simulink model "TEST_C___MAPD"  (R2015b)
settings: Solver=ode23tb  StartTime=0.0  StopTime=1  RelTol=1e-3
InitFcn:
  | eps=1e-10
  | 
  | Lg=90e-6;
  | l=100e-6; r=2e-3;
  | tff=10e-6;
  | w=2*pi*60;
  | z_lead =966.3602;
  | p_lead =5.6324e+03;
  | Vdc=2000;
undefined symbols (not defined in the file or in its folder): C, magnitude
libraries: powerlib x26, powerlib_meascontrol x12, simulink x8, simulink_extras x3
settings Model: Creator=Shahed Mortazavian  LastModifiedBy=Masoud
settings DataIOCC: SaveFormat=Array  SignalLoggingSaveFormat=ModelDataLogs
settings OptimizationCC: ExpressionDepthLimit=2147483647
settings DebuggingCC: UnderspecifiedInitializationDetection=Classic  MergeDetectMultiDrivingBlocksExec=none  SolverPrmCheckMsg=warning  FcnCallInpInsideContextMsg=UseLocalSettings  StateNameClashWarn=warning
settings HardwareCC: ProdBitPerPointer=32  ProdLargestAtomicFloat=None  ProdIntDivRoundTo=Undefined  ProdEndianess=Unspecified  ProdWordSize=32  ProdHWDeviceType=32-bit Generic
settings GRTTargetCC: GeneratePreprocessorConditionals=Disable all  CombineOutputUpdateFcns=off  GRTInterface=on
settings ConfigComp: CovModelRefEnable=Off  CovSFcnEnable=off

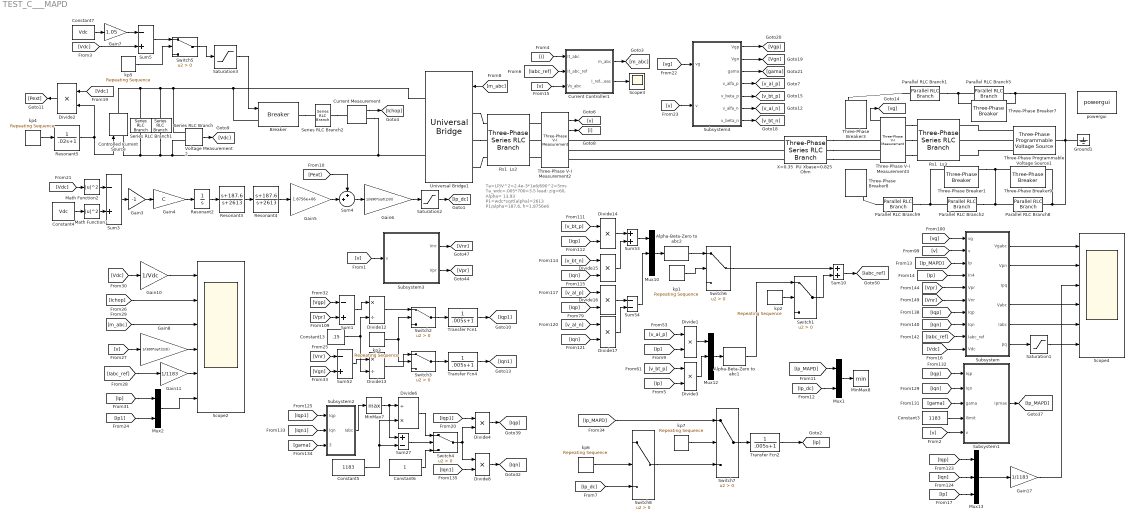
== system TEST_C___MAPD ==
  note: Ta=LP/V^2=2.4e-3*1e6/690^2=5ms
      | Ta_wdc=.005*700=3.5
      | lead: zig=60, Alpha= 13.93
      | P1=wdc*sqrt(alpha)=2613
      | P1/alpha=187.6, h=1.8756e6
  Alpha-Beta-Zero to abc1 : powerlib_meascontrol/Transformations/Alpha-Beta-Zero to abc
  Alpha-Beta-Zero to abc2 : powerlib_meascontrol/Transformations/Alpha-Beta-Zero to abc
  Breaker : powerlib/Elements/Breaker  InitialState=0  SwitchingTimes="[1/60  5/60]"  External=on  BreakerResistance=0.01  SnubberResistance=1e6  SnubberCapacitance=inf  Measurements=None  MoreParameters=on  NoBreakLoop=off
  Constant13 : Constant  Value=.15
  Constant3 : Constant  Value=1183
  Constant4 : Constant  Value=Vdc
  Constant5 : Constant  Value=1183
  Constant6 : Constant
  Constant7 : Constant  Value=Vdc
  Controlled Current Source : powerlib/Electrical Sources/Controlled Current Source  Initialize=on  Source_Type=AC  Amplitude=0  Phase=0  Frequency=0  Measurements=None
  Current Controller1 : Subsystem
  Current Measurement : powerlib/Measurements/Current Measurement  PhasorSimulation=off  OutputType=Complex  PSBequivalent=0
  Divide{1..4,8,14..17} (9 alike) : Product  Inputs=**
  Divide12 : Product  Inputs=*/
  Divide13 : Product  Inputs=*/
  Divide6 : Product  Inputs=/*
  Gain10 : Gain  Gain=1/Vdc
  Gain11 : Gain  Gain=1/1183
  Gain17 : Gain  Gain=1/1183
  Gain3 : Gain  Gain=-1
  Gain4 : Gain  Gain=C
  Gain5 : Gain  Gain=1.8756e+06
  Gain6 : Gain  Gain=1/(690*sqrt(2/3))
  Gain7 : Gain  Gain=1.05
  Gain8 : Gain  Gain=1/(690*sqrt(2/3))
  Ground1 : powerlib/Elements/Ground  LConnTagsString=a
  Math Function1 : Math  Operator=magnitude^2  SaturateOnIntegerOverflow=on
  Math Function2 : Math  Operator=magnitude^2  SaturateOnIntegerOverflow=on
  MinMax7 : MinMax  Function=max
  MinMax8 : MinMax
  Mux1 : Mux  Inputs=2
  Mux10 : Mux  Inputs=3
  Mux12 : Mux  Inputs=3
  Mux13 : Mux  Inputs=3
  Mux2 : Mux  Inputs=2
  Parallel RLC Branch1 : powerlib/Elements/Parallel RLC Branch  LConnTagsString=a  RConnTagsString=__new0  BranchType=R  Resistance=1e-3  Inductance=1e-3  SetiL0=off  InitialCurrent=0  Capacitance=1e-6  Setx0=off  InitialVoltage=0  Measurements=None
  Parallel RLC Branch2 : powerlib/Elements/Parallel RLC Branch  LConnTagsString=a  RConnTagsString=__new0  BranchType=R  Resistance=1e-3  Inductance=1e-3  SetiL0=off  InitialCurrent=0  Capacitance=1e-6  Setx0=off  InitialVoltage=0  Measurements=None
  Parallel RLC Branch5 : powerlib/Elements/Parallel RLC Branch  LConnTagsString=a  RConnTagsString=__new0  BranchType=R  Resistance=.3e-3  Inductance=1e-3  SetiL0=off  InitialCurrent=0  Capacitance=1e-6  Setx0=off  InitialVoltage=0  Measurements=None
  Parallel RLC Branch8 : powerlib/Elements/Parallel RLC Branch  LConnTagsString=a  RConnTagsString=__new0  BranchType=R  Resistance=1e-3  Inductance=1e-3  SetiL0=off  InitialCurrent=0  Capacitance=1e-6  Setx0=off  InitialVoltage=0  Measurements=None
  Parallel RLC Branch9 : powerlib/Elements/Parallel RLC Branch  LConnTagsString=a  RConnTagsString=__new0  BranchType=R  Resistance=2e-3  Inductance=1e-3  SetiL0=off  InitialCurrent=0  Capacitance=1e-6  Setx0=off  InitialVoltage=0  Measurements=None
  Resonant2 : TransferFcn  Denominator=[1 0 ]
  Resonant3 : TransferFcn  Numerator=[1 187.6]  Denominator=[1 2613]
  Resonant4 : TransferFcn  Numerator=[1 187.6]  Denominator=[1 2613]
  Resonant5 : TransferFcn  Denominator=[.02 1]
  Rs1  Ls2 : powerlib/Elements/Three-Phase Series RLC Branch  LConnTagsString=A|B|C  RConnTagsString=A|B|C  BranchType=RL  Resistance=r  Inductance=l  Capacitance=1e-6  Measurements=None
  Rs1  Ls3 : powerlib/Elements/Three-Phase Series RLC Branch  LConnTagsString=A|B|C  RConnTagsString=A|B|C  BranchType=R  Resistance=1e-3  Inductance=l  Capacitance=1e-6  Measurements=None
  Saturation1 : Saturate  UpperLimit=1.5  LowerLimit=-.5
  Saturation2 : Saturate  UpperLimit=2000  LowerLimit=0
  Saturation3 : Saturate  UpperLimit=1000  LowerLimit=0
  Scope2 : Scope  NumInputPorts=6
  Scope3 : Scope
  Scope4 : Scope  NumInputPorts=6
  Series RLC Branch : powerlib/Elements/Series RLC Branch  LConnTagsString=__new0  RConnTagsString=__new0  BranchType=C  Resistance=1  Inductance=1e-3  SetiL0=off  InitialCurrent=0  Capacitance=C*2  Setx0=on  InitialVoltage=Vdc  Measurements=None
  Series RLC Branch1 : powerlib/Elements/Series RLC Branch  LConnTagsString=__new0  RConnTagsString=__new0  BranchType=R  Resistance=1e10  Inductance=1e-3  SetiL0=off  InitialCurrent=0  Capacitance=C  Setx0=on  InitialVoltage=2500  Measurements=None
  Series RLC Branch2 : powerlib/Elements/Series RLC Branch  LConnTagsString=__new0  RConnTagsString=__new0  BranchType=R  Resistance=1  Inductance=1e-3  SetiL0=off  InitialCurrent=0  Capacitance=C  Setx0=on  InitialVoltage=2500  Measurements=None
  Subsystem : Subsystem
  Subsystem1 : Subsystem
  Subsystem2 : Subsystem
  Subsystem3 : Subsystem
  Subsystem4 : Subsystem
  Sum{1,3,5,52} (4 alike) : Sum  Inputs=-+
  Sum10 : Sum
  Sum27 : Sum  Inputs=+-
  Sum4 : Sum  Inputs=++|
  Sum53 : Sum
  Sum54 : Sum  Inputs=--
  Switch{1..8} (8 alike) : Switch  Criteria=u2 > Threshold
  Three-Phase Programmable Voltage Source1 : powerlib/Electrical Sources/Three-Phase Programmable Voltage Source  PositiveSequence=[690 0 60]  VariationEntity=Amplitude  VariationType=Table of time-amplitude pairs  VariationTypeAlt=Step  VariationStep=0.5  VariationRate=10  VariationMagnitude=0.3  VariationFrequency=2  VariationTiming=[1 2]  VariationPhaseA=on  Amplitudes=[1 1 .61 .61]  TimeValues=[0 .3 .30001 10]  HarmonicGeneration=off  HarmonicA=[3 0.2 -25 0]  HarmonicB=[2 0.15 35 2]  Timing="[0.05  3]"  BusType=swing  Pref=0  Qref=0  Qmin=-inf  Qmax=inf
  Three-Phase V-I Measurement2 : powerlib/Measurements/Three-Phase V-I Measurement  VoltageMeasurement=phase-to-ground  SetLabelV=off  LabelV=Vabc  Vpu=off  VpuLL=off  CurrentMeasurement=yes  SetLabelI=off  LabelI=Iabc  Ipu=off  Pbase=100e6  Vbase=500e3  OutputType=Complex  PhasorSimulation=off  PSBequivalent=0
  Three-Phase V-I Measurement3 : powerlib/Measurements/Three-Phase V-I Measurement  VoltageMeasurement=phase-to-ground  SetLabelV=off  LabelV=Vabc  Vpu=off  VpuLL=off  CurrentMeasurement=yes  SetLabelI=off  LabelI=Iabc  Ipu=off  Pbase=100e6  Vbase=500e3  OutputType=Complex  PhasorSimulation=off  PSBequivalent=0
  Three-Phase Breaker1 : powerlib/Elements/Three-Phase Breaker  InitialState=open  SwitchA=on  SwitchB=on  SwitchC=on  SwitchTimes=.6  External=off  BreakerResistance=1e-40  SnubberResistance=1e6  SnubberCapacitance=inf  Measurements=None
  Three-Phase Breaker3 : powerlib/Elements/Three-Phase Breaker  InitialState=open  SwitchA=on  SwitchB=on  SwitchC=on  SwitchTimes=.3  External=off  BreakerResistance=1e-40  SnubberResistance=1e6  SnubberCapacitance=inf  Measurements=None
  Three-Phase Breaker7 : powerlib/Elements/Three-Phase Breaker  InitialState=open  SwitchA=on  SwitchB=on  SwitchC=on  SwitchTimes=.5  External=off  BreakerResistance=1e-40  SnubberResistance=1e6  SnubberCapacitance=inf  Measurements=None
  Three-Phase Breaker8 : powerlib/Elements/Three-Phase Breaker  InitialState=open  SwitchA=on  SwitchB=on  SwitchC=on  SwitchTimes=.2  External=off  BreakerResistance=1e-40  SnubberResistance=1e6  SnubberCapacitance=inf  Measurements=None
  Three-Phase Breaker9 : powerlib/Elements/Three-Phase Breaker  InitialState=open  SwitchA=on  SwitchB=on  SwitchC=on  SwitchTimes=.6  External=off  BreakerResistance=1e-40  SnubberResistance=1e6  SnubberCapacitance=inf  Measurements=None
  Transfer Fcn1 : TransferFcn  Numerator=1  Denominator=[.005 1]
  Transfer Fcn2 : TransferFcn  Numerator=1  Denominator=[.005 1]
  Transfer Fcn4 : TransferFcn  Numerator=1  Denominator=[.005 1]
  Universal Bridge1 : powerlib/Power Electronics/Universal Bridge  Arms=3  SnubberResistance=1e5  SnubberCapacitance=inf  Device=Average-model based VSC  Ron=1e-3  Lon=0  ForwardVoltages="[  0  0  ]"  ForwardVoltage=0  GTOparameters=[ 10e-6 , 20e-6 ]  IGBTparameters=[ 1e-6 , 2e-6 ]  Measurements=None  Measurements_2=None  converterType=Rectifier
  Voltage Measurement2 : powerlib/Measurements/Voltage Measurement  PhasorSimulation=off  OutputType=Complex  PSBequivalent=0
  X=0.35  PU Xbase=0.825  Ohm : powerlib/Elements/Three-Phase Series RLC Branch  LConnTagsString=A|B|C  RConnTagsString=A|B|C  BranchType=L  Resistance=.0001  Inductance=.15/377  Capacitance=1e-6  Measurements=None
  kp1 : simulink/Sources/Repeating Sequence  rep_seq_t=[0 .3 .3+eps 10]  rep_seq_y=[0 0 1 1]
  kp2 : simulink/Sources/Repeating Sequence  rep_seq_t=[0 .03 .03+eps 10]  rep_seq_y=[0 0 1 1]
  kp3 : simulink/Sources/Repeating Sequence  rep_seq_t=[0 .31 .31+eps 10]  rep_seq_y=[0 0 1 1]
  kp4 : simulink/Sources/Repeating Sequence  rep_seq_t=[0 .02 .02+eps 10]  rep_seq_y=3/2*400*[0 0 .8 .8]
  kp5 : simulink/Sources/Repeating Sequence  rep_seq_t=[0 .3 .3+eps 10]  rep_seq_y=[0 0 1 1]
  kp6 : simulink/Sources/Repeating Sequence  rep_seq_t=[0 .5 .5+eps 10]  rep_seq_y=[0 0 1 1]
  kp7 : simulink/Sources/Repeating Sequence  rep_seq_t=[0 .7 .7+eps 10]  rep_seq_y=[0 0 1 1]
  powergui : powerlib/powergui  Priority=2  SimulationMode=Discrete  SolverType=Tustin  SampleTime=5e-5  frequency=60  SPID=off  DisableSnubberDevices=off  DisableRonSwitches=off  DisableVfSwitches=off  SwTol=0  DisplayEquations=off  Interpol=off  ExternalGateDelay=off  methode=off  Ts=0  FunctionMessages=off  echomessages=off  HookPort=off  EnableUseOfTLC=off  x0status=blocks  frequencyindice=0  Pbase=100e6  ErrMax=1e-4  Iterations=50  UnitsV=kV  UnitsW=MW  buscounter=0  RestoreLinks=warning  ResistiveCurrentMeasurement=off  Frange=[0:2:500]  Ylog=off  Xlog=on  ShowGrid=off  save=off  variable=ZData  structure=Data  ZoomFFT=off  StartTime=.22  cycles=2  DisplayStyle=1  fundamental=60  FreqAxis=off  MaxFrequency=1000  frequencyindicesteady=1  RmsSteady=1  display=off
  wires:
  [i] -> Current Controller1/1(It_abc)
  [v] -> Current Controller1/3(Vs_abc)
  Current Controller1/1(m_abc) -> [m_abc]
  [Iabc_ref] -> Current Controller1/2(It_abc_ref)
  Current Controller1/2(I_ref_meas) -> Scope3/1
  Divide14/1 -> Sum53/1
  Divide15/1 -> Sum53/2
  Divide16/1 -> Sum54/1
  Divide17/1 -> Sum54/2
  Mux10/1 -> Alpha-Beta-Zero to abc2/1
  Sum53/1 -> Mux10/1
  Sum54/1 -> Mux10/2
  [v_bt_p] -> Divide14/1
  [Iqp] -> Divide14/2
  [v_bt_n] -> Divide15/1
  [Iqn] -> Divide15/2
  [v_al_p] -> Divide16/1
  [Iqp] -> Divide16/2
  [v_al_n] -> Divide17/1
  [Iqn] -> Divide17/2
  [gama] -> Subsystem1/3(gama)
  Constant3/1 -> Subsystem1/4(Ilimit)
  [Iqp] -> Subsystem1/1(Iqp)
  [Iqn] -> Subsystem1/2(Iqn)
  [Ip] -> Divide1/2
  [v_bt_p] -> Divide3/1
  [Ip] -> Divide3/2
  Mux12/1 -> Alpha-Beta-Zero to abc1/1
  Divide1/1 -> Mux12/1
  Divide3/1 -> Mux12/2
  [v_al_p] -> Divide1/1
  Alpha-Beta-Zero to abc2/1 -> Switch6/1
  kp1/1 -> Switch6/2
  Switch6/1 -> Sum10/1
  [Iqp1] -> Subsystem2/1(Iqp)
  [Iqn1] -> Subsystem2/2(Iqn)
  [gama] -> Subsystem2/3(gama)
  Constant5/1 -> Divide6/2, Sum27/2
  Subsystem2/1(Iabc) -> MinMax7/1
  Sum27/1 -> Switch4/2
  MinMax7/1 -> Divide6/1, Sum27/1
  Divide6/1 -> Switch4/1
  Constant6/1 -> Switch4/3
  Switch4/1 -> Divide4/2, Divide8/1
  [Iqp1] -> Divide4/1
  Divide4/1 -> [Iqp]
  [Iqn1] -> Divide8/2
  Divide8/1 -> [Iqn]
  Three-Phase V-I Measurement3/1 -> [vg]
  [vg] -> Subsystem/1(vg)
  [v] -> Subsystem/2(v)
  [Vpr] -> Subsystem/5(Vpr)
  [Vnr] -> Subsystem/6(Vnr)
  [Iqp] -> Subsystem/7(Iqp)
  [Iqn] -> Subsystem/8(Iqn)
  [Iabc_ref] -> Subsystem/9(Iabc_ref)
  Subsystem/2(Vpn) -> Scope4/2
  Subsystem/4(Vabc) -> Scope4/4
  Subsystem/5(Iabc) -> Scope4/5
  Subsystem/6(pq) -> Saturation1/1
  Subsystem3/2(Vpr) -> [Vpr]
  Subsystem3/1(Vnr) -> [Vnr]
  [v] -> Subsystem3/1(v)
  Alpha-Beta-Zero to abc1/1 -> Switch1/1
  [v] -> Subsystem1/5(v)
  Subsystem/1(Vgabc) -> Scope4/1
  Sum10/1 -> [Iabc_ref]
  kp2/1 -> Switch1/2
  Switch1/1 -> Sum10/2
  Subsystem1/1(Ipmax) -> [Ip_MAPD]
  [Ip_MAPD] -> Subsystem/3(Ip)
  Three-Phase V-I Measurement2/1 -> [v]
  Three-Phase V-I Measurement2/2 -> [i]
  [m_abc] -> Universal Bridge1/1
  kp4/1 -> Resonant5/1
  Voltage Measurement2/1 -> [Vdc]
  [Vdc] -> Divide2/1
  Divide2/1 -> [Pext]
  Resonant5/1 -> Divide2/2, Controlled Current Source/1
  [Vdc] -> Math Function2/1
  Constant4/1 -> Math Function1/1
  Math Function2/1 -> Sum3/1
  Math Function1/1 -> Sum3/2
  Sum3/1 -> Gain3/1
  Gain3/1 -> Gain4/1
  Gain4/1 -> Resonant2/1
  Resonant2/1 -> Resonant3/1
  Resonant3/1 -> Resonant4/1
  Resonant4/1 -> Gain5/1
  Gain5/1 -> Sum4/2
  [Pext] -> Sum4/1
  Sum4/1 -> Gain6/1
  Gain6/1 -> Saturation2/1
  Saturation2/1 -> [Ip_dc]
  Mux1/1 -> MinMax8/1
  [Ip_MAPD] -> Mux1/1
  [Ip_dc] -> Mux1/2
  [Ip] -> Subsystem/4(In4)
  Saturation1/1 -> Scope4/6
  [Vdc] -> Subsystem/10(Vdc)
  Mux13/1 -> Gain17/1
  Gain17/1 -> Scope4/3
  [Iqp] -> Mux13/1
  [Iqn] -> Mux13/2
  [Ip] -> Mux13/3
  [vg] -> Subsystem4/1(vg)
  [v] -> Subsystem4/2(v)
  Subsystem4/1(Vgp) -> [Vgp]
  Subsystem4/2(Vgn) -> [Vgn]
  Subsystem4/3(gama) -> [gama]
  Subsystem4/4(v_alfa_p) -> [v_al_p]
  Subsystem4/5(v_beta_p) -> [v_bt_p]
  Subsystem4/6(v_alfa_n) -> [v_al_n]
  Subsystem4/7(v_beta_n) -> [v_bt_n]
  Constant7/1 -> Gain7/1
  Gain7/1 -> Sum5/1
  Sum5/1 -> Switch5/1
  kp5/1 -> Switch5/2
  [Vdc] -> Sum5/2
  Switch5/1 -> Saturation3/1
  Current Measurement/1 -> [Ichop]
  Saturation3/1 -> Breaker/1
  [Vdc] -> Gain10/1
  [v] -> Gain8/1
  [Iabc_ref] -> Gain11/1
  [m_abc] -> Scope2/3
  Gain8/1 -> Scope2/4
  Gain10/1 -> Scope2/1
  Gain11/1 -> Scope2/5
  [Ip1] -> Mux2/2
  [Ip] -> Mux2/1
  Mux2/1 -> Scope2/6
  [Ichop] -> Scope2/2
  Sum1/1 -> Divide12/1
  Divide12/1 -> Switch2/1
  Sum52/1 -> Divide13/1
  Divide13/1 -> Switch3/1
  kp3/1 -> Switch2/2, Switch3/2
  Switch2/1 -> Transfer Fcn1/1
  Switch3/1 -> Transfer Fcn4/1
  [Vgn] -> Sum52/2
  [Vpr] -> Sum1/2
  [Vnr] -> Sum52/1
  Transfer Fcn1/1 -> [Iqp1]
  Transfer Fcn4/1 -> [Iqn1]
  [Vgp] -> Sum1/1
  Constant13/1 -> Divide12/2, Divide13/2
  Switch7/1 -> Transfer Fcn2/1
  Transfer Fcn2/1 -> [Ip]
  Switch8/1 -> Switch7/3
  [Ip_dc] -> Switch8/3
  kp6/1 -> Switch8/2
  [Ip_MAPD] -> Switch7/1
  kp7/1 -> Switch7/2
  connections:
  X=0.35  PU Xbase=0.825  Ohm/RConn2 -- Three-Phase V-I Measurement3/RConn2
  X=0.35  PU Xbase=0.825  Ohm/RConn3 -- Three-Phase V-I Measurement3/RConn3
  Parallel RLC Branch5/LConn1 -- Three-Phase Breaker7/LConn1 -- Parallel RLC Branch1/RConn1
  Parallel RLC Branch8/LConn1 -- Parallel RLC Branch2/RConn1 -- Three-Phase Breaker1/RConn1 -- Three-Phase Breaker9/LConn1
  Parallel RLC Branch5/RConn1 -- Three-Phase Breaker7/RConn1 -- Parallel RLC Branch8/RConn1 -- Three-Phase Breaker9/RConn1 -- Three-Phase Programmable Voltage Source1/LConn1 -- Ground1/LConn1
  Three-Phase V-I Measurement3/LConn2 -- Rs1  Ls3/LConn2
  Parallel RLC Branch1/LConn1 -- Three-Phase Breaker3/RConn1
  Three-Phase Programmable Voltage Source1/RConn2 -- Rs1  Ls3/RConn2
  Three-Phase Programmable Voltage Source1/RConn3 -- Rs1  Ls3/RConn3
  Parallel RLC Branch9/LConn1 -- Three-Phase Breaker8/RConn1
  X=0.35  PU Xbase=0.825  Ohm/RConn1 -- Three-Phase V-I Measurement3/RConn1
  Three-Phase Programmable Voltage Source1/RConn1 -- Rs1  Ls3/RConn1
  Three-Phase V-I Measurement3/LConn3 -- Rs1  Ls3/LConn3
  Three-Phase V-I Measurement3/LConn1 -- Rs1  Ls3/LConn1
  Parallel RLC Branch9/RConn1 -- Parallel RLC Branch2/LConn1 -- Three-Phase Breaker1/LConn1
  Voltage Measurement2/LConn2 -- Current Measurement/RConn1 -- Universal Bridge1/RConn2 -- Series RLC Branch/RConn1 -- Controlled Current Source/LConn1 -- Series RLC Branch1/RConn1
  X=0.35  PU Xbase=0.825  Ohm/LConn3 -- Three-Phase V-I Measurement2/RConn3
  Three-Phase V-I Measurement2/LConn2 -- Rs1  Ls2/RConn2
  Universal Bridge1/LConn2 -- Rs1  Ls2/LConn2
  Universal Bridge1/LConn3 -- Rs1  Ls2/LConn3
  Series RLC Branch1/LConn1 -- Controlled Current Source/RConn1 -- Series RLC Branch/LConn1 -- Breaker/LConn1 -- Universal Bridge1/RConn1 -- Voltage Measurement2/LConn1
  Three-Phase V-I Measurement2/LConn3 -- Rs1  Ls2/RConn3
  Universal Bridge1/LConn1 -- Rs1  Ls2/LConn1
  X=0.35  PU Xbase=0.825  Ohm/LConn1 -- Three-Phase V-I Measurement2/RConn1
  Three-Phase V-I Measurement2/LConn1 -- Rs1  Ls2/RConn1
  X=0.35  PU Xbase=0.825  Ohm/LConn2 -- Three-Phase V-I Measurement2/RConn2
  Breaker/RConn1 -- Series RLC Branch2/LConn1
  Series RLC Branch2/RConn1 -- Current Measurement/LConn1

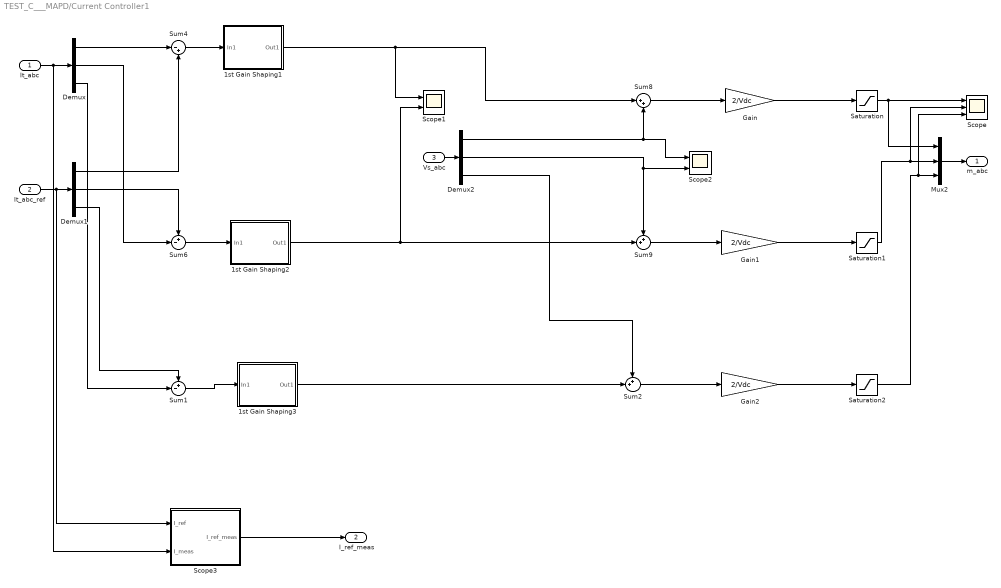
== system TEST_C___MAPD/Current Controller1 ==
  It_abc : Inport
  It_abc_ref : Inport  Port=2
  Vs_abc : Inport  Port=3
  1st Gain Shaping1 : Subsystem
  1st Gain Shaping2 : Subsystem
  1st Gain Shaping3 : Subsystem
  Demux : Demux  Outputs=3
  Demux1 : Demux  Outputs=3
  Demux2 : Demux  Outputs=3
  Gain : Gain  Gain=2/Vdc
  Gain1 : Gain  Gain=2/Vdc
  Gain2 : Gain  Gain=2/Vdc
  Mux2 : Mux  Inputs=3
  Saturation : Saturate  UpperLimit=1  LowerLimit=-1
  Saturation1 : Saturate  UpperLimit=1  LowerLimit=-1
  Saturation2 : Saturate  UpperLimit=1  LowerLimit=-1
  Scope : Scope  NumInputPorts=3
  Scope1 : Scope  NumInputPorts=2
  Scope2 : Scope  NumInputPorts=2
  Scope3 : Subsystem
  Sum1 : Sum  Inputs=+-|
  Sum2 : Sum  Inputs=++|
  Sum4 : Sum  Inputs=|-+
  Sum6 : Sum  Inputs=+-|
  Sum8 : Sum  Inputs=|++
  Sum9 : Sum  Inputs=++|
  m_abc : Outport
  I_ref_meas : Outport  Port=2
  wires:
  Demux2/1 -> Scope2/1, Sum8/2
  Demux2/2 -> Scope2/2, Sum9/1
  Sum6/1 -> 1st Gain Shaping2/1(In1)
  It_abc/1 -> Scope3/2(I_meas), Demux/1
  It_abc_ref/1 -> Scope3/1(I_ref), Demux1/1
  Vs_abc/1 -> Demux2/1
  Sum8/1 -> Gain/1
  Sum9/1 -> Gain1/1
  Mux2/1 -> m_abc/1
  Gain/1 -> Saturation/1
  Gain1/1 -> Saturation1/1
  Saturation2/1 -> Scope/3, Mux2/3
  Saturation/1 -> Scope/1, Mux2/1
  Saturation1/1 -> Mux2/2, Scope/2
  Demux1/1 -> Sum4/2
  Demux/1 -> Sum4/1
  Sum4/1 -> 1st Gain Shaping1/1(In1)
  Demux1/2 -> Sum6/1
  Demux/2 -> Sum6/2
  Demux1/3 -> Sum1/1
  Demux/3 -> Sum1/2
  Sum1/1 -> 1st Gain Shaping3/1(In1)
  Gain2/1 -> Saturation2/1
  Sum2/1 -> Gain2/1
  Demux2/3 -> Sum2/1
  1st Gain Shaping2/1(Out1) -> Scope1/2, Sum9/2
  1st Gain Shaping3/1(Out1) -> Sum2/2
  1st Gain Shaping1/1(Out1) -> Scope1/1, Sum8/1
  Scope3/1(I_ref_meas) -> I_ref_meas/1

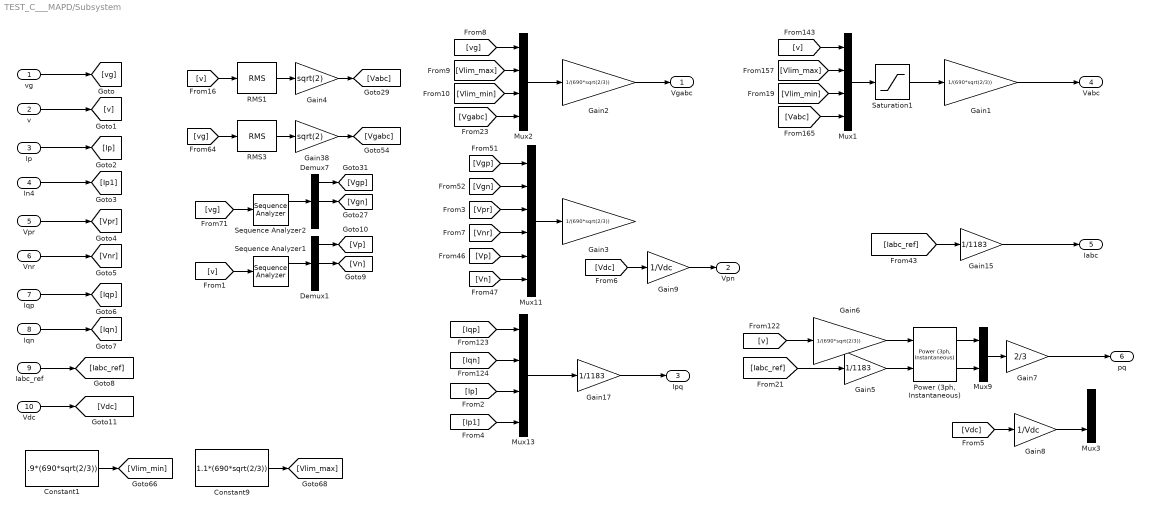
== system TEST_C___MAPD/Subsystem ==
  vg : Inport
  v : Inport  Port=2
  Ip : Inport  Port=3
  In4 : Inport  Port=4
  Vpr : Inport  Port=5
  Vnr : Inport  Port=6
  Iqp : Inport  Port=7
  Iqn : Inport  Port=8
  Iabc_ref : Inport  Port=9
  Vdc : Inport  Port=10
  Constant1 : Constant  Value=.9*(690*sqrt(2/3))
  Constant9 : Constant  Value=1.1*(690*sqrt(2/3))
  Demux1 : Demux  Outputs=3
  Demux7 : Demux  Outputs=3
  Gain{1..3,6} (4 alike) : Gain  Gain=1/(690*sqrt(2/3))
  Gain15 : Gain  Gain=1/1183
  Gain17 : Gain  Gain=1/1183
  Gain38 : Gain  Gain=sqrt(2)
  Gain4 : Gain  Gain=sqrt(2)
  Gain5 : Gain  Gain=1/1183
  Gain7 : Gain  Gain=2/3
  Gain8 : Gain  Gain=1/Vdc
  Gain9 : Gain  Gain=1/Vdc
  Mux1 : Mux
  Mux11 : Mux  Inputs=6
  Mux13 : Mux
  Mux2 : Mux
  Mux3 : Mux  Inputs=2
  Mux9 : Mux  Inputs=2
  "Power (3ph, Instantaneous)" : powerlib_meascontrol/Measurements/Power (3ph, Instantaneous)
  RMS1 : powerlib_meascontrol/Measurements/RMS  TrueRMS=on  Freq=60  RMSInit=0  Ts=0
  RMS3 : powerlib_meascontrol/Measurements/RMS  TrueRMS=on  Freq=60  RMSInit=0  Ts=0
  Saturation1 : Saturate  UpperLimit=800  LowerLimit=-800
  Sequence Analyzer1 : powerlib_meascontrol/Measurements/Sequence Analyzer  Freq=60  n=1  seq=Positive Negative Zero  InInit=[1, 0]  Ts=0
  Sequence Analyzer2 : powerlib_meascontrol/Measurements/Sequence Analyzer  Freq=60  n=1  seq=Positive Negative Zero  InInit=[1, 0]  Ts=0
  Vgabc : Outport
  Vpn : Outport  Port=2
  Ipq : Outport  Port=3
  Vabc : Outport  Port=4
  Iabc : Outport  Port=5
  pq : Outport  Port=6
  wires:
  vg/1 -> [vg]
  v/1 -> [v]
  Vpr/1 -> [Vpr]
  Vnr/1 -> [Vnr]
  Iqp/1 -> [Iqp]
  Iqn/1 -> [Iqn]
  Iabc_ref/1 -> [Iabc_ref]
  [Vp] -> Mux11/5
  [Vn] -> Mux11/6
  [Vgp] -> Mux11/1
  [Vgn] -> Mux11/2
  Mux11/1 -> Gain3/1
  Mux2/1 -> Gain2/1
  Mux1/1 -> Saturation1/1
  [Vpr] -> Mux11/3
  [Vnr] -> Mux11/4
  [Vlim_max] -> Mux2/2
  [Vlim_min] -> Mux2/3
  [Vgabc] -> Mux2/4
  [vg] -> Mux2/1
  [Vlim_max] -> Mux1/2
  [Vlim_min] -> Mux1/3
  [Vabc] -> Mux1/4
  [v] -> Mux1/1
  "Power (3ph, Instantaneous)"/2 -> Mux9/2
  "Power (3ph, Instantaneous)"/1 -> Mux9/1
  [Iabc_ref] -> Gain5/1
  [v] -> Gain6/1
  Mux13/1 -> Gain17/1
  Gain17/1 -> Ipq/1
  [Iqp] -> Mux13/1
  [Iqn] -> Mux13/2
  [Iabc_ref] -> Gain15/1
  RMS3/1 -> Gain38/1
  [vg] -> RMS3/1
  Gain38/1 -> [Vgabc]
  RMS1/1 -> Gain4/1
  [v] -> RMS1/1
  Gain4/1 -> [Vabc]
  Gain2/1 -> Vgabc/1
  Gain1/1 -> Vabc/1
  Saturation1/1 -> Gain1/1
  Gain15/1 -> Iabc/1
  Mux9/1 -> Gain7/1
  [vg] -> Sequence Analyzer2/1
  Sequence Analyzer2/1 -> Demux7/1
  Demux7/1 -> [Vgp]
  Demux7/2 -> [Vgn]
  [v] -> Sequence Analyzer1/1
  Sequence Analyzer1/1 -> Demux1/1
  Demux1/1 -> [Vp]
  Demux1/2 -> [Vn]
  Constant1/1 -> [Vlim_min]
  Constant9/1 -> [Vlim_max]
  Gain5/1 -> "Power (3ph, Instantaneous)"/2
  Gain6/1 -> "Power (3ph, Instantaneous)"/1
  Ip/1 -> [Ip]
  [Ip] -> Mux13/3
  In4/1 -> [Ip1]
  [Ip1] -> Mux13/4
  Vdc/1 -> [Vdc]
  [Vdc] -> Gain8/1
  Gain8/1 -> Mux3/2
  [Vdc] -> Gain9/1
  Gain9/1 -> Vpn/1
  Gain7/1 -> pq/1

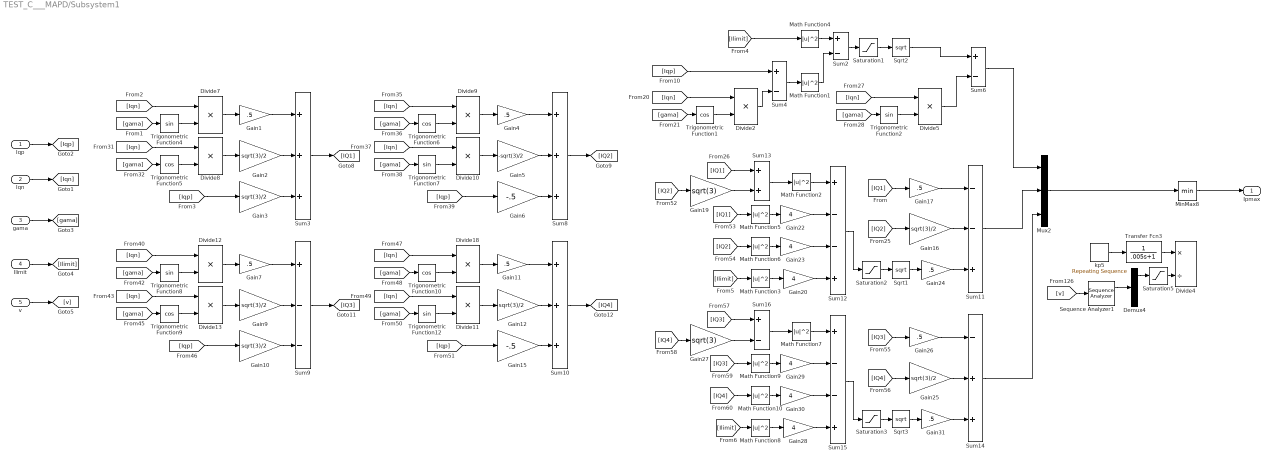
== system TEST_C___MAPD/Subsystem1 ==
  Iqp : Inport
  Iqn : Inport  Port=2
  gama : Inport  Port=3
  Ilimit : Inport  Port=4
  v : Inport  Port=5
  Demux4 : Demux  Outputs=3
  Divide{2,5,7..13,18} (10 alike) : Product  Inputs=**
  Divide4 : Product  Inputs=*/
  Gain{1,4,7,11,17,24,26,31} (8 alike) : Gain  Gain=.5
  Gain{2..3,9..10,12,16,25} (7 alike) : Gain  Gain=sqrt(3)/2
  Gain15 : Gain  Gain=-.5
  Gain19 : Gain  Gain=sqrt(3)
  Gain{20,22..23,28..30} (6 alike) : Gain  Gain=4
  Gain27 : Gain  Gain=sqrt(3)
  Gain5 : Gain  Gain=-sqrt(3)/2
  Gain6 : Gain  Gain=-.5
  Math Function{1..10} (10 alike) : Math  Operator=magnitude^2  SaturateOnIntegerOverflow=on
  MinMax8 : MinMax
  Mux2 : Mux  Inputs=3
  Saturation1 : Saturate  UpperLimit=10000000  LowerLimit=1
  Saturation2 : Saturate  UpperLimit=10000000  LowerLimit=1
  Saturation3 : Saturate  UpperLimit=10000000  LowerLimit=1
  Saturation5 : Saturate  UpperLimit=1000  LowerLimit=10
  Sequence Analyzer1 : powerlib_meascontrol/Measurements/Sequence Analyzer  Freq=60  n=1  seq=Positive Negative Zero  InInit=[1, 0]  Ts=0
  Sqrt1 : Sqrt  SaturateOnIntegerOverflow=on
  Sqrt2 : Sqrt  SaturateOnIntegerOverflow=on
  Sqrt3 : Sqrt  SaturateOnIntegerOverflow=on
  Sum10 : Sum  Inputs=+++
  Sum11 : Sum  Inputs=--+
  Sum12 : Sum  Inputs=+--+
  Sum13 : Sum
  Sum14 : Sum  Inputs=-++
  Sum15 : Sum  Inputs=+--+
  Sum{2,4,6,16} (4 alike) : Sum  Inputs=+-
  Sum3 : Sum  Inputs=+++
  Sum8 : Sum  Inputs=+++
  Sum9 : Sum  Inputs=+--
  Transfer Fcn3 : TransferFcn  Numerator=1  Denominator=[.005 1]
  Trigonometric Function{1,5..6,9..10} (5 alike) : Trigonometry  Operator=cos
  Trigonometric Function{2,4,7..8,12} (5 alike) : Trigonometry
  kp5 : simulink/Sources/Repeating Sequence  rep_seq_t=[0 .05 .05+eps 10]  rep_seq_y=6e5*(2/3)*[0 0 1 1]
  Ipmax : Outport
  wires:
  [Iqp] -> Sum4/1
  Sum4/1 -> Math Function1/1
  Gain3/1 -> Sum3/3
  Sum3/1 -> [IQ1]
  [gama] -> Trigonometric Function6/1
  Gain6/1 -> Sum8/3
  Sum8/1 -> [IQ2]
  [Iqn] -> Divide9/1
  Gain5/1 -> Sum8/2
  [Iqn] -> Divide10/1
  [gama] -> Trigonometric Function7/1
  Divide10/1 -> Gain5/1
  Trigonometric Function6/1 -> Divide9/2
  Divide9/1 -> Gain4/1
  [Iqp] -> Gain6/1
  Trigonometric Function7/1 -> Divide10/2
  Gain4/1 -> Sum8/1
  Sum9/1 -> [IQ3]
  [Iqn] -> Divide18/1
  [gama] -> Trigonometric Function10/1
  Divide11/1 -> Gain12/1
  Trigonometric Function9/1 -> Divide13/2
  Sum10/1 -> [IQ4]
  [gama] -> Trigonometric Function9/1
  Gain9/1 -> Sum9/2
  [Iqn] -> Divide12/1
  Trigonometric Function8/1 -> Divide12/2
  Trigonometric Function10/1 -> Divide18/2
  Gain11/1 -> Sum10/1
  [gama] -> Trigonometric Function8/1
  [Iqn] -> Divide11/1
  Divide13/1 -> Gain9/1
  [Iqp] -> Gain15/1
  Gain10/1 -> Sum9/3
  Divide18/1 -> Gain11/1
  [Iqn] -> Divide13/1
  Gain12/1 -> Sum10/2
  Gain7/1 -> Sum9/1
  Divide12/1 -> Gain7/1
  Trigonometric Function12/1 -> Divide11/2
  [gama] -> Trigonometric Function12/1
  Gain15/1 -> Sum10/3
  [Iqp] -> Gain10/1
  Divide7/1 -> Gain1/1
  [gama] -> Trigonometric Function1/1
  [Iqn] -> Divide2/1
  Divide2/1 -> Sum4/2
  Trigonometric Function1/1 -> Divide2/2
  Gain24/1 -> Sum11/3
  Math Function1/1 -> Sum2/2
  Gain22/1 -> Sum12/2
  Iqn/1 -> [Iqn]
  Iqp/1 -> [Iqp]
  Trigonometric Function4/1 -> Divide7/2
  Trigonometric Function5/1 -> Divide8/2
  Divide8/1 -> Gain2/1
  [gama] -> Trigonometric Function5/1
  Gain1/1 -> Sum3/1
  [Iqn] -> Divide8/1
  Gain2/1 -> Sum3/2
  Sum12/1 -> Saturation2/1
  [Iqn] -> Divide5/1
  Trigonometric Function2/1 -> Divide5/2
  [gama] -> Trigonometric Function2/1
  Sum6/1 -> Mux2/1
  Sum14/1 -> Mux2/3
  Sum11/1 -> Mux2/2
  Divide5/1 -> Sum6/2
  Sqrt2/1 -> Sum6/1
  [Ilimit] -> Math Function4/1
  Math Function4/1 -> Sum2/1
  Sum2/1 -> Saturation1/1
  Saturation1/1 -> Sqrt2/1
  Math Function2/1 -> Sum12/1
  Gain19/1 -> Sum13/2
  Saturation2/1 -> Sqrt1/1
  Sqrt1/1 -> Gain24/1
  Sqrt3/1 -> Gain31/1
  [IQ3] -> Gain26/1
  Math Function8/1 -> Gain28/1
  Math Function7/1 -> Sum15/1
  Gain25/1 -> Sum14/2
  Gain28/1 -> Sum15/4
  [IQ3] -> Math Function9/1
  [IQ4] -> Math Function10/1
  [IQ4] -> Gain25/1
  Saturation3/1 -> Sqrt3/1
  Math Function9/1 -> Gain29/1
  Gain29/1 -> Sum15/2
  Gain26/1 -> Sum14/1
  Gain31/1 -> Sum14/3
  Math Function10/1 -> Gain30/1
  Gain27/1 -> Sum16/2
  Gain30/1 -> Sum15/3
  Sum15/1 -> Saturation3/1
  Sum16/1 -> Math Function7/1
  [IQ4] -> Gain27/1
  [IQ3] -> Sum16/1
  [Ilimit] -> Math Function3/1
  Math Function3/1 -> Gain20/1
  Gain17/1 -> Sum11/1
  [IQ1] -> Math Function5/1
  Math Function5/1 -> Gain22/1
  Gain20/1 -> Sum12/4
  [IQ1] -> Sum13/1
  Math Function6/1 -> Gain23/1
  Gain23/1 -> Sum12/3
  [IQ2] -> Math Function6/1
  Sum13/1 -> Math Function2/1
  [IQ2] -> Gain19/1
  [IQ2] -> Gain16/1
  [IQ1] -> Gain17/1
  Gain16/1 -> Sum11/2
  gama/1 -> [gama]
  [gama] -> Trigonometric Function4/1
  [Iqn] -> Divide7/1
  [Iqp] -> Gain3/1
  Ilimit/1 -> [Ilimit]
  [Ilimit] -> Math Function8/1
  Mux2/1 -> MinMax8/1
  [v] -> Sequence Analyzer1/1
  Sequence Analyzer1/1 -> Demux4/1
  Demux4/1 -> Saturation5/1
  kp5/1 -> Transfer Fcn3/1
  Transfer Fcn3/1 -> Divide4/1
  Saturation5/1 -> Divide4/2
  MinMax8/1 -> Ipmax/1
  v/1 -> [v]

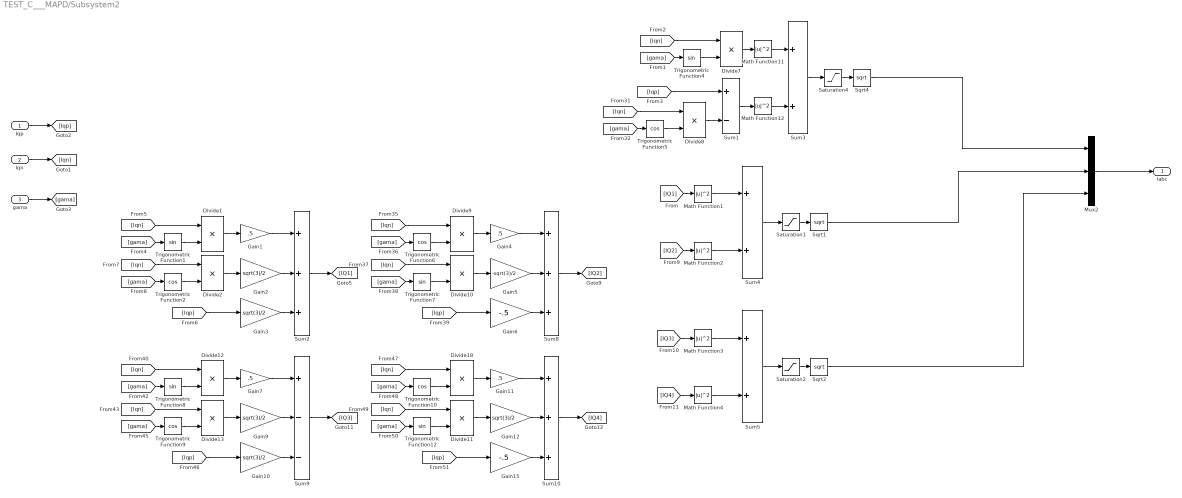
== system TEST_C___MAPD/Subsystem2 ==
  Iqp : Inport
  Iqn : Inport  Port=2
  gama : Inport  Port=3
  Divide{1..2,7..13,18} (10 alike) : Product  Inputs=**
  Gain{1,4,7,11} (4 alike) : Gain  Gain=.5
  Gain{2..3,9..10,12} (5 alike) : Gain  Gain=sqrt(3)/2
  Gain15 : Gain  Gain=-.5
  Gain5 : Gain  Gain=-sqrt(3)/2
  Gain6 : Gain  Gain=-.5
  Math Function{1..4,11..12} (6 alike) : Math  Operator=magnitude^2  SaturateOnIntegerOverflow=on
  Mux2 : Mux  Inputs=3
  Saturation1 : Saturate  UpperLimit=10000000  LowerLimit=1
  Saturation2 : Saturate  UpperLimit=10000000  LowerLimit=1
  Saturation4 : Saturate  UpperLimit=10000000  LowerLimit=1
  Sqrt1 : Sqrt  SaturateOnIntegerOverflow=on
  Sqrt2 : Sqrt  SaturateOnIntegerOverflow=on
  Sqrt4 : Sqrt  SaturateOnIntegerOverflow=on
  Sum1 : Sum  Inputs=+-
  Sum10 : Sum  Inputs=+++
  Sum2 : Sum  Inputs=+++
  Sum3 : Sum
  Sum4 : Sum
  Sum5 : Sum
  Sum8 : Sum  Inputs=+++
  Sum9 : Sum  Inputs=+--
  Trigonometric Function{1,4,7..8,12} (5 alike) : Trigonometry
  Trigonometric Function{2,5..6,9..10} (5 alike) : Trigonometry  Operator=cos
  Iabc : Outport
  wires:
  [Iqp] -> Sum1/1
  [Iqn] -> Divide7/1
  [gama] -> Trigonometric Function4/1
  gama/1 -> [gama]
  Mux2/1 -> Iabc/1
  [Iqn] -> Divide8/1
  Divide7/1 -> Math Function11/1
  [gama] -> Trigonometric Function5/1
  Divide8/1 -> Sum1/2
  Trigonometric Function5/1 -> Divide8/2
  Trigonometric Function4/1 -> Divide7/2
  Iqp/1 -> [Iqp]
  Iqn/1 -> [Iqn]
  Math Function11/1 -> Sum3/1
  Sum1/1 -> Math Function12/1
  Math Function12/1 -> Sum3/2
  Saturation4/1 -> Sqrt4/1
  Sqrt4/1 -> Mux2/1
  Sum3/1 -> Saturation4/1
  Gain3/1 -> Sum2/3
  Sum2/1 -> [IQ1]
  [gama] -> Trigonometric Function6/1
  Gain6/1 -> Sum8/3
  Sum8/1 -> [IQ2]
  [Iqn] -> Divide9/1
  Gain5/1 -> Sum8/2
  [Iqn] -> Divide10/1
  [gama] -> Trigonometric Function7/1
  Divide10/1 -> Gain5/1
  Trigonometric Function6/1 -> Divide9/2
  Divide9/1 -> Gain4/1
  [Iqp] -> Gain6/1
  Trigonometric Function7/1 -> Divide10/2
  Gain4/1 -> Sum8/1
  Sum9/1 -> [IQ3]
  [Iqn] -> Divide18/1
  [gama] -> Trigonometric Function10/1
  Divide11/1 -> Gain12/1
  Trigonometric Function9/1 -> Divide13/2
  Sum10/1 -> [IQ4]
  [gama] -> Trigonometric Function9/1
  Gain9/1 -> Sum9/2
  [Iqn] -> Divide12/1
  Trigonometric Function8/1 -> Divide12/2
  Trigonometric Function10/1 -> Divide18/2
  Gain11/1 -> Sum10/1
  [gama] -> Trigonometric Function8/1
  [Iqn] -> Divide11/1
  Divide13/1 -> Gain9/1
  [Iqp] -> Gain15/1
  Gain10/1 -> Sum9/3
  Divide18/1 -> Gain11/1
  [Iqn] -> Divide13/1
  Gain12/1 -> Sum10/2
  Gain7/1 -> Sum9/1
  Divide12/1 -> Gain7/1
  Trigonometric Function12/1 -> Divide11/2
  [gama] -> Trigonometric Function12/1
  Gain15/1 -> Sum10/3
  [Iqp] -> Gain10/1
  Divide1/1 -> Gain1/1
  Trigonometric Function1/1 -> Divide1/2
  Trigonometric Function2/1 -> Divide2/2
  Divide2/1 -> Gain2/1
  [gama] -> Trigonometric Function2/1
  Gain1/1 -> Sum2/1
  [Iqn] -> Divide2/1
  Gain2/1 -> Sum2/2
  [gama] -> Trigonometric Function1/1
  [Iqn] -> Divide1/1
  [Iqp] -> Gain3/1
  [IQ1] -> Math Function1/1
  Math Function1/1 -> Sum4/1
  [IQ2] -> Math Function2/1
  Math Function2/1 -> Sum4/2
  Saturation1/1 -> Sqrt1/1
  Sum4/1 -> Saturation1/1
  [IQ3] -> Math Function3/1
  Math Function3/1 -> Sum5/1
  [IQ4] -> Math Function4/1
  Math Function4/1 -> Sum5/2
  Saturation2/1 -> Sqrt2/1
  Sum5/1 -> Saturation2/1
  Sqrt1/1 -> Mux2/2
  Sqrt2/1 -> Mux2/3

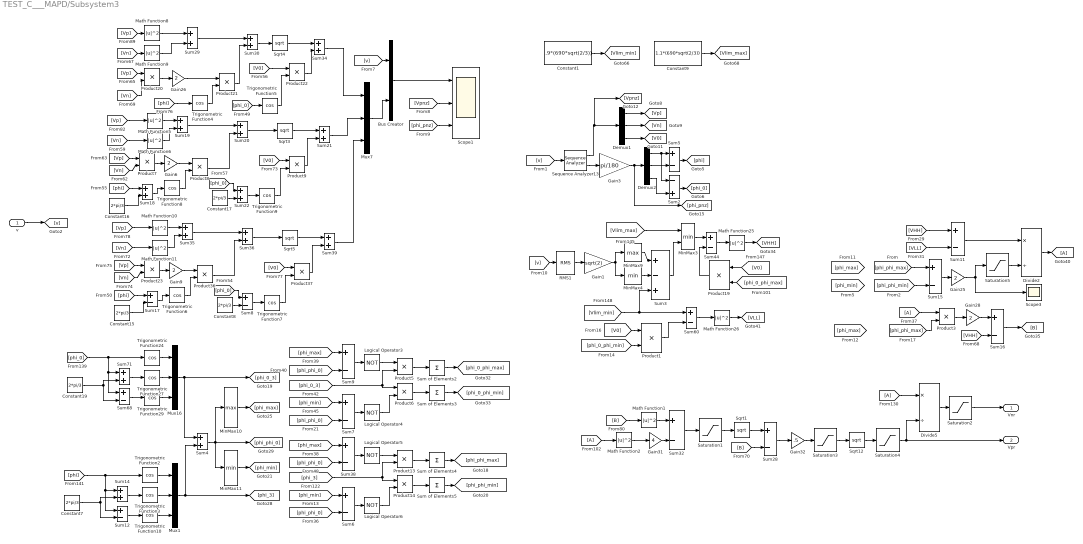
== system TEST_C___MAPD/Subsystem3 ==
  v : Inport
  Bus Creator : BusCreator  Inputs=2
  Constant1 : Constant  Value=.9*(690*sqrt(2/3))
  Constant{7..8,15..17,19} (6 alike) : Constant  Value=2*pi/3
  Constant9 : Constant  Value=1.1*(690*sqrt(2/3))
  Demux1 : Demux  Outputs=3
  Demux2 : Demux  Outputs=3
  Divide2 : Product  Inputs=*/
  Divide5 : Product  Inputs=*/
  Gain1 : Gain  Gain=sqrt(2)
  Gain{6,9,25..26,28} (5 alike) : Gain  Gain=2
  Gain3 : Gain  Gain=pi/180
  Gain31 : Gain  Gain=4
  Gain32 : Gain  Gain=.5
  Logical Operator{3..6} (4 alike) : Logic  Operator=NOT  AllPortsSameDT=off  OutDataTypeStr=boolean
  Math Function{1..2,5..6,8..11,25..26} (10 alike) : Math  Operator=magnitude^2  SaturateOnIntegerOverflow=on
  MinMax10 : MinMax  Function=max
  MinMax11 : MinMax
  MinMax3 : MinMax  Inputs=2
  MinMax4 : MinMax
  MinMax9 : MinMax  Function=max
  Mux1 : Mux  Inputs=3
  Mux16 : Mux  Inputs=3
  Mux7 : Mux  Inputs=3
  Product{1,3,5..9,13..14,19..23,36..37} (16 alike) : Product
  RMS1 : powerlib_meascontrol/Measurements/RMS  TrueRMS=on  Freq=60  RMSInit=0  Ts=0
  Saturation1 : Saturate  UpperLimit=1e16  LowerLimit=0
  Saturation2 : Saturate  UpperLimit=.4*690*sqrt(2/3)  LowerLimit=0
  Saturation3 : Saturate  UpperLimit=1e16  LowerLimit=0
  Saturation4 : Saturate  UpperLimit=1.2*690*sqrt(2/3)  LowerLimit=10
  Saturation5 : Saturate  UpperLimit=100  LowerLimit=0.1
  Scope1 : Scope  NumInputPorts=3
  Scope3 : Scope
  Sequence Analyzer13 : powerlib_meascontrol/Measurements/Sequence Analyzer  Freq=60  n=1  seq=Positive Negative Zero  InInit=[1, 0]  Ts=0
  Sqrt{1,3..5,12} (5 alike) : Sqrt  SaturateOnIntegerOverflow=on
  Sum of Elements{2..5} (4 alike) : Sum  Inputs=+
  Sum{5..9,11..12,15..17,28,32,38,44,60,68} (16 alike) : Sum  Inputs=+-
  Sum{4,14,18..22,29..30,34..36,39,71} (14 alike) : Sum
  Sum2 : Sum  Inputs=-+
  Sum3 : Sum  Inputs=+-+
  Trigonometric Function{2..10,24,27,29} (12 alike) : Trigonometry  Operator=cos
  Vnr : Outport
  Vpr : Outport  Port=2
  wires:
  Math Function6/1 -> Sum19/2
  [phi] -> Sum18/1
  Sum21/1 -> Mux7/2
  Constant17/1 -> Sum22/2
  Sum20/1 -> Sqrt3/1
  Product7/1 -> Gain6/1
  Sum2/1 -> [phi_0]
  Constant16/1 -> Sum18/2
  Sum19/1 -> Sum20/1
  Demux1/3 -> [V0]
  Product9/1 -> Sum21/2
  Sum5/1 -> [phi]
  [v] -> Bus Creator/1
  Demux2/3 -> Sum2/2
  Bus Creator/1 -> Scope1/1
  [Vp] -> Product7/1
  Mux7/1 -> Bus Creator/2
  Sequence Analyzer13/1 -> [Vpnz], Demux1/1
  Demux1/2 -> [Vn]
  Sum22/1 -> Trigonometric Function9/1
  Demux1/1 -> [Vp]
  Sqrt3/1 -> Sum21/1
  [Vn] -> Math Function6/1
  Sum18/1 -> Trigonometric Function8/1
  [Vpnz] -> Scope1/2
  [Vp] -> Math Function5/1
  [phi_pnz] -> Scope1/3
  Trigonometric Function8/1 -> Product8/2
  Sum34/1 -> Mux7/1
  Sum39/1 -> Mux7/3
  [phi_0] -> Sum22/1
  Sum14/1 -> Trigonometric Function3/1
  Product5/1 -> Sum of Elements2/1
  [phi] -> Trigonometric Function2/1, Sum14/1, Sum12/1
  Sum71/1 -> Trigonometric Function27/1
  [v] -> RMS1/1
  Product6/1 -> Sum of Elements3/1
  Sum68/1 -> Trigonometric Function29/1
  Trigonometric Function27/1 -> Mux16/2
  Gain1/1 -> MinMax4/1, MinMax9/1
  Sum3/1 -> MinMax3/2
  Sum9/1 -> Logical Operator3/1
  MinMax9/1 -> Sum3/1
  MinMax3/1 -> Sum44/1
  [phi_0] -> Sum68/1, Sum71/1, Trigonometric Function24/1
  Trigonometric Function2/1 -> Mux1/1
  Trigonometric Function3/1 -> Mux1/2
  Mux1/1 -> [phi_3], Sum4/2
  Mux16/1 -> [phi_0_3], Sum4/1
  Constant19/1 -> Sum71/2, Sum68/2
  MinMax11/1 -> [phi_min]
  MinMax10/1 -> [phi_max]
  Sum7/1 -> Logical Operator4/1
  MinMax4/1 -> Sum3/2
  RMS1/1 -> Gain1/1
  Trigonometric Function24/1 -> Mux16/1
  Sum12/1 -> Trigonometric Function10/1
  Trigonometric Function10/1 -> Mux1/3
  [phi_max] -> Sum9/1
  [phi_phi_0] -> Sum9/2
  Trigonometric Function29/1 -> Mux16/3
  Constant7/1 -> Sum12/2, Sum14/2
  Product14/1 -> Sum of Elements5/1
  Logical Operator5/1 -> Product13/1
  Product19/1 -> Sum44/2
  [phi_0_phi_min] -> Product1/2
  Sum of Elements4/1 -> [phi_phi_max]
  [phi_phi_0] -> Sum7/2
  Sum4/1 -> [phi_phi_0], MinMax10/1, MinMax11/1
  [phi_min] -> Sum7/1
  Sum6/1 -> Logical Operator6/1
  [phi_phi_0] -> Sum6/2
  [phi_3] -> Product13/2, Product14/1
  [V0] -> Product19/1
  [phi_0_phi_max] -> Product19/2
  Sum of Elements3/1 -> [phi_0_phi_min]
  Logical Operator3/1 -> Product5/1
  [V0] -> Product1/1
  Product1/1 -> Sum60/2
  [phi_max] -> Sum38/1
  Sum38/1 -> Logical Operator5/1
  Product13/1 -> Sum of Elements4/1
  Logical Operator4/1 -> Product6/2
  [phi_0_3] -> Product6/1, Product5/2
  Sum of Elements2/1 -> [phi_0_phi_max]
  [phi_min] -> Sum6/1
  Sum of Elements5/1 -> [phi_phi_min]
  [phi_phi_0] -> Sum38/2
  [Vlim_min] -> Sum3/3, Sum60/1
  Logical Operator6/1 -> Product14/2
  [phi_phi_max] -> Sum15/1
  [phi_phi_min] -> Sum15/2
  Saturation3/1 -> Sqrt12/1
  [phi_phi_max] -> Product3/2
  Sqrt12/1 -> Saturation4/1
  [VHH] -> Sum16/2
  [B] -> Sum28/2
  Math Function1/1 -> Sum32/1
  Math Function2/1 -> Gain31/1
  Product3/1 -> Gain28/1
  Saturation4/1 -> Vpr/1, Divide5/2
  Math Function25/1 -> [VHH]
  Sqrt1/1 -> Sum28/1
  [VLL] -> Sum11/2
  [A] -> Math Function2/1
  Gain28/1 -> Sum16/1
  Sum60/1 -> Math Function26/1
  [B] -> Math Function1/1
  Math Function26/1 -> [VLL]
  Sum32/1 -> Saturation1/1
  [A] -> Product3/1
  Gain32/1 -> Saturation3/1
  Sum44/1 -> Math Function25/1
  Sum16/1 -> [B]
  Sum11/1 -> Divide2/1
  Sum15/1 -> Gain25/1
  [A] -> Divide5/1
  [Vlim_max] -> MinMax3/1
  [VHH] -> Sum11/1
  Gain31/1 -> Sum32/2
  Saturation1/1 -> Sqrt1/1
  Divide5/1 -> Saturation2/1
  Sum28/1 -> Gain32/1
  Gain3/1 -> [phi_pnz], Demux2/1
  Demux2/2 -> Sum5/2
  Demux2/1 -> Sum2/1, Sum5/1
  Sequence Analyzer13/2 -> Gain3/1
  [v] -> Sequence Analyzer13/1
  Divide2/1 -> [A]
  Gain9/1 -> Product36/1
  Product36/1 -> Sum36/2
  [Vn] -> Product23/2
  Sqrt5/1 -> Sum39/1
  [Vp] -> Product23/1
  Sum35/1 -> Sum36/1
  Math Function11/1 -> Sum35/2
  Math Function10/1 -> Sum35/1
  Trigonometric Function7/1 -> Product37/2
  Sum36/1 -> Sqrt5/1
  [Vn] -> Math Function11/1
  Product37/1 -> Sum39/2
  [V0] -> Product37/1
  Product23/1 -> Gain9/1
  Sum30/1 -> Sqrt4/1
  Product22/1 -> Sum34/2
  [phi_0] -> Sum8/1
  Product20/1 -> Gain26/1
  Sum29/1 -> Sum30/1
  [phi] -> Sum17/1
  [Vn] -> Math Function9/1
  Math Function8/1 -> Sum29/1
  [V0] -> Product22/1
  [Vn] -> Product7/2
  Trigonometric Function4/1 -> Product21/2
  Product21/1 -> Sum30/2
  [Vp] -> Math Function8/1
  Sum17/1 -> Trigonometric Function6/1
  Math Function9/1 -> Sum29/2
  Trigonometric Function5/1 -> Product22/2
  Sum8/1 -> Trigonometric Function7/1
  [phi] -> Trigonometric Function4/1
  Gain26/1 -> Product21/1
  Math Function5/1 -> Sum19/1
  Product8/1 -> Sum20/2
  [Vn] -> Product20/2
  Constant15/1 -> Sum17/2
  Trigonometric Function9/1 -> Product9/2
  Constant8/1 -> Sum8/2
  Gain6/1 -> Product8/1
  Trigonometric Function6/1 -> Product36/2
  Sqrt4/1 -> Sum34/1
  [Vp] -> Product20/1
  [Vp] -> Math Function10/1
  [phi_0] -> Trigonometric Function5/1
  [V0] -> Product9/1
  Saturation2/1 -> Vnr/1
  v/1 -> [v]
  Constant1/1 -> [Vlim_min]
  Constant9/1 -> [Vlim_max]
  Saturation5/1 -> Divide2/2
  Gain25/1 -> Scope3/1, Saturation5/1

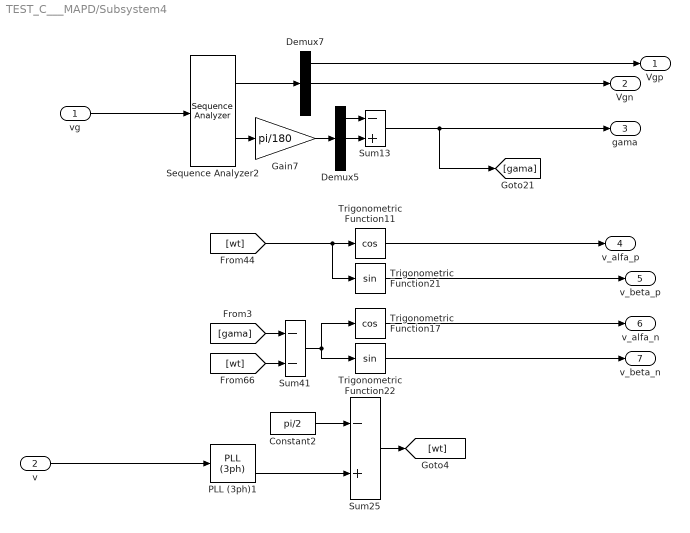
== system TEST_C___MAPD/Subsystem4 ==
  vg : Inport
  v : Inport  Port=2
  Constant2 : Constant  Value=pi/2
  Demux5 : Demux  Outputs=3
  Demux7 : Demux  Outputs=3
  Gain7 : Gain  Gain=pi/180
  PLL (3ph)1 : powerlib_meascontrol/PLL/PLL (3ph)  Fmin=45  Par_Init=[0, 60]  ParK=[180, 3200, 1]  TcD=1e-4  MaxRateChangeFreq=12  FilterCutOffFreq=25  Ts=0  AGC=on
  Sequence Analyzer2 : powerlib_meascontrol/Measurements/Sequence Analyzer  Freq=60  n=1  seq=Positive Negative Zero  InInit=[1, 0]  Ts=0
  Sum13 : Sum  Inputs=-+
  Sum25 : Sum  Inputs=-+
  Sum41 : Sum  Inputs=--
  Trigonometric Function11 : Trigonometry  Operator=cos
  Trigonometric Function17 : Trigonometry  Operator=cos
  Trigonometric Function21 : Trigonometry
  Trigonometric Function22 : Trigonometry
  Vgp : Outport
  Vgn : Outport  Port=2
  gama : Outport  Port=3
  v_alfa_p : Outport  Port=4
  v_beta_p : Outport  Port=5
  v_alfa_n : Outport  Port=6
  v_beta_n : Outport  Port=7
  wires:
  v/1 -> PLL (3ph)1/1
  Sum25/1 -> [wt]
  Demux5/1 -> Sum13/1
  Sum13/1 -> [gama], gama/1
  Demux5/2 -> Sum13/2
  PLL (3ph)1/2 -> Sum25/2
  Constant2/1 -> Sum25/1
  Demux7/1 -> Vgp/1
  Sequence Analyzer2/2 -> Gain7/1
  vg/1 -> Sequence Analyzer2/1
  Gain7/1 -> Demux5/1
  Sequence Analyzer2/1 -> Demux7/1
  Demux7/2 -> Vgn/1
  [wt] -> Trigonometric Function21/1, Trigonometric Function11/1
  [wt] -> Sum41/2
  Sum41/1 -> Trigonometric Function17/1, Trigonometric Function22/1
  Trigonometric Function17/1 -> v_alfa_n/1
  Trigonometric Function11/1 -> v_alfa_p/1
  Trigonometric Function22/1 -> v_beta_n/1
  Trigonometric Function21/1 -> v_beta_p/1
  [gama] -> Sum41/1

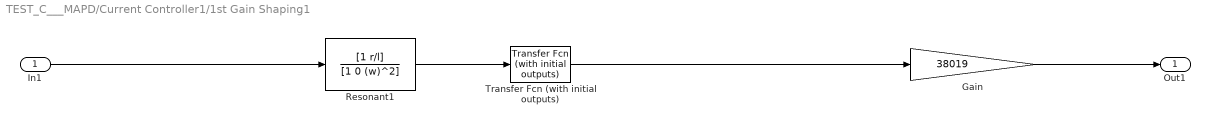
== system TEST_C___MAPD/Current Controller1/1st Gain Shaping1 ==
  In1 : Inport
  Gain : Gain  Gain=38019
  Resonant1 : TransferFcn  Numerator=[1 r/l]  Denominator=[1 0 (w)^2]
  Transfer Fcn (with initial outputs) : simulink_extras/Additional Linear/Transfer Fcn (with initial outputs)  N=[1 5205]  D=[1 30340]  Y0=0  U0=0
  Out1 : Outport
  wires:
  Resonant1/1 -> Transfer Fcn (with initial outputs)/1
  In1/1 -> Resonant1/1
  Gain/1 -> Out1/1
  Transfer Fcn (with initial outputs)/1 -> Gain/1

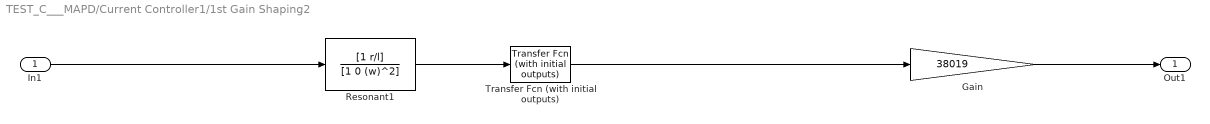
== system TEST_C___MAPD/Current Controller1/1st Gain Shaping2 ==
  In1 : Inport
  Gain : Gain  Gain=38019
  Resonant1 : TransferFcn  Numerator=[1 r/l]  Denominator=[1 0 (w)^2]
  Transfer Fcn (with initial outputs) : simulink_extras/Additional Linear/Transfer Fcn (with initial outputs)  N=[1 5205]  D=[1 30340]  Y0=0  U0=0
  Out1 : Outport
  wires:
  Transfer Fcn (with initial outputs)/1 -> Gain/1
  Gain/1 -> Out1/1
  In1/1 -> Resonant1/1
  Resonant1/1 -> Transfer Fcn (with initial outputs)/1

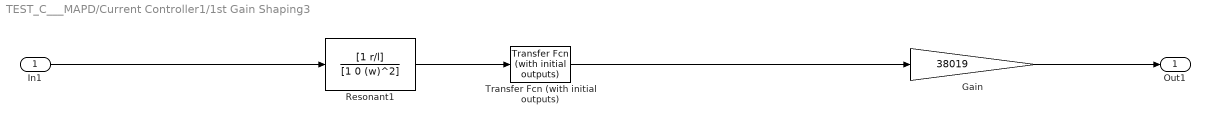
== system TEST_C___MAPD/Current Controller1/1st Gain Shaping3 ==
  In1 : Inport
  Gain : Gain  Gain=38019
  Resonant1 : TransferFcn  Numerator=[1 r/l]  Denominator=[1 0 (w)^2]
  Transfer Fcn (with initial outputs) : simulink_extras/Additional Linear/Transfer Fcn (with initial outputs)  N=[1 5205]  D=[1 30340]  Y0=0  U0=0
  Out1 : Outport
  wires:
  Resonant1/1 -> Transfer Fcn (with initial outputs)/1
  In1/1 -> Resonant1/1
  Gain/1 -> Out1/1
  Transfer Fcn (with initial outputs)/1 -> Gain/1

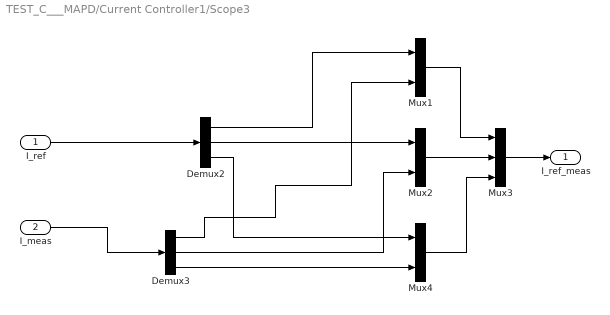
== system TEST_C___MAPD/Current Controller1/Scope3 ==
  I_ref : Inport
  I_meas : Inport  Port=2
  Demux2 : Demux  Outputs=3
  Demux3 : Demux  Outputs=3
  Mux1 : Mux  Inputs=2
  Mux2 : Mux  Inputs=2
  Mux3 : Mux  Inputs=3
  Mux4 : Mux  Inputs=2
  I_ref_meas : Outport
  wires:
  I_meas/1 -> Demux3/1
  I_ref/1 -> Demux2/1
  Demux2/1 -> Mux1/1
  Demux3/1 -> Mux1/2
  Mux1/1 -> Mux3/1
  Demux2/2 -> Mux2/1
  Demux3/2 -> Mux2/2
  Mux2/1 -> Mux3/2
  Demux2/3 -> Mux4/1
  Demux3/3 -> Mux4/2
  Mux4/1 -> Mux3/3
  Mux3/1 -> I_ref_meas/1
